simulink model "QAM16"  (R2024a)
settings: Solver=ode45  StartTime=0.0  StopTime=5000  RelTol=1e-3  EnableMultiTasking=on
PreLoadFcn:
  | QAM16_PreLoadFcn
values from neighbouring files (symbols this model uses):
  chan = [1+j*0.1 .2 j*0.2 0 0 0 0 0 0 0]    [QAM16_PreLoadFcn.m]
  hh = sinc(-3:.25:3)    [QAM16_PreLoadFcn.m]
  k = 9    [QAM16_PreLoadFcn.m]
  k_i0 = (4*theta_0*theta_0)/(1+2*eta*theta_0+theta_0*theta_0)    [QAM16_PreLoadFcn.m]
  k_p0 = (4*eta*theta_0)/(1+2*eta*theta_0+theta_0*theta_0)    [QAM16_PreLoadFcn.m]
  mu = 0.004    [QAM16_PreLoadFcn.m]
undefined symbols (not defined in the file or in its folder): j, QAM, S, vsva2197, xcvc1902, xlipgetpartsetting
libraries: hdlBasic x260, dspmlti4 x2, hdlUtilities x1, hdlDSPIP x1, simulink x1, vmcUtilities x1
(part 2 of 3)

== system QAM16/DUT/Carrier Recovery/DPLL Loop Filter ==
  phs_err : Inport
  KI : hdlBasic/Constant  Priority=5  const=k_i0  gui_display_data_type=Fixed-point  arith_type=Signed (2's comp)  n_bits=16  bin_pt=15  preci_type=Single  exp_width=8  frac_width=24  explicit_period=on  period=4  XmcBlockStatus=1  maskContainerNames=tabcontainer1  block_type=constant  block_config=sysgen:Constant_config
  KP : hdlBasic/Constant  Priority=5  const=k_p0  gui_display_data_type=Fixed-point  arith_type=Signed (2's comp)  n_bits=16  bin_pt=15  preci_type=Single  exp_width=8  frac_width=24  explicit_period=on  period=4  XmcBlockStatus=1  maskContainerNames=tabcontainer1  block_type=constant  block_config=sysgen:Constant_config
  MPY KI : hdlBasic/Mult  precision=User Defined  arith_type="Signed  (2's comp)"  n_bits=32  bin_pt=28  quantization=Truncate  overflow=Wrap  en=off  latency=0  opt_float=off  fp_mult_usage=No Usage  use_behavioral_HDL=off  opt=Speed  use_embedded=on  optimum_pipeline=off  pipeline=off  use_rpm=off  placement_style=Rectangular shape  XmcBlockStatus=1  maskContainerNames=group1  block_type=mult  block_config=sysgen:Mult_config  block_width=598  block_height=876
  MPY KP : hdlBasic/Mult  precision=User Defined  arith_type="Signed  (2's comp)"  n_bits=32  bin_pt=28  quantization=Truncate  overflow=Wrap  en=off  latency=0  opt_float=off  fp_mult_usage=No Usage  use_behavioral_HDL=off  opt=Speed  use_embedded=on  optimum_pipeline=off  pipeline=off  use_rpm=off  placement_style=Rectangular shape  XmcBlockStatus=1  maskContainerNames=group1  block_type=mult  block_config=sysgen:Mult_config  block_width=598  block_height=876
  addsub : hdlBasic/AddSub  mode=Addition  use_carryin=off  use_carryout=off  en=off  latency=0  precision=User Defined  arith_type=Unsigned  n_bits=10  bin_pt=10  quantization=Truncate  overflow=Wrap  use_behavioral_HDL=on  hw_selection=Fabric  pipelined=off  use_rpm=off  XmcBlockStatus=1  maskContainerNames=tabcontainer1  block_type=addsub  block_config=sysgen:Addsub_config
  addsub1 : hdlBasic/AddSub  mode=Addition  use_carryin=off  use_carryout=off  en=off  latency=0  precision=User Defined  arith_type="Signed  (2's comp)"  n_bits=32  bin_pt=28  quantization="Round  (unbiased: +/- Inf)"  overflow=Wrap  use_behavioral_HDL=on  hw_selection=Fabric  pipelined=off  use_rpm=off  XmcBlockStatus=1  maskContainerNames=tabcontainer1  block_type=addsub  block_config=sysgen:Addsub_config
  register : hdlBasic/Register  init=0  rst=off  en=off  XmcBlockStatus=1  maskContainerNames=tabcontainer1  block_type=register  block_config=sysgen:Register_config
  y : Outport  VectorParamsAs1DForOutWhenUnconnected=off
  wires:
  KI/1 -> MPY KI/2
  KP/1 -> MPY KP/2
  MPY KI/1 -> addsub1/1
  phs_err/1 -> MPY KI/1, MPY KP/1
  register/1 -> addsub1/2
  addsub1/1 -> addsub/2, register/1
  MPY KP/1 -> addsub/1
  addsub/1 -> y/1

== system QAM16/DUT/Carrier Recovery/Phase Detector ==
  note: The slicer circuit consistis primarily of several
      | comparators and a small look-up table.
  note: The arctangent operation is performed using
      | a custom CORDIC processor.
  I_in : Inport
  Q_in : Inport  Port=2
  Constant : hdlBasic/Constant  const=0  gui_display_data_type=Fixed-point  arith_type=Signed (2's comp)  n_bits=1  bin_pt=0  preci_type=Single  exp_width=8  frac_width=24  explicit_period=off  period=1  XmcBlockStatus=1  maskContainerNames=tabcontainer1  block_type=constant  block_config=sysgen:Constant_config
  Cordic : Subsystem
  NegB_Cmplx Mult : Subsystem
  Slicer : Subsystem
  Terminator : Terminator
  Terminator1 : Terminator
  det_I : Outport  VectorParamsAs1DForOutWhenUnconnected=off
  det_Q : Outport  Port=2  VectorParamsAs1DForOutWhenUnconnected=off
  phs_err : Outport  Port=3  VectorParamsAs1DForOutWhenUnconnected=off
  wires:
  NegB_Cmplx Mult/1(p_r) -> Cordic/1(x)
  Cordic/3(z_n) -> phs_err/1
  Constant/1 -> Cordic/3(z)
  Cordic/1(x_n) -> Terminator/1
  Cordic/2(y_n) -> Terminator1/1
  NegB_Cmplx Mult/2(p_i) -> Cordic/2(y)
  Slicer/2(det_Q) -> NegB_Cmplx Mult/2(a_i), det_Q/1
  Slicer/1(det_ I) -> NegB_Cmplx Mult/1(a_r), det_I/1
  Q_in/1 -> Slicer/2(Q_in), NegB_Cmplx Mult/4(b_i)
  I_in/1 -> Slicer/1(I_in), NegB_Cmplx Mult/3(b_r)

== system QAM16/16-QAM Data Shaping & Interpolation/QAM16 Source/QAM16 - I/Random Integer Generator ==
  Rounding Function : Rounding  Operator=round
  Uniform Random Number : UniformRandomNumber  Minimum=-0.49  Maximum=M-1 + 0.49  Seed=seed  SampleTime=Ts
  Out1 : Outport  VectorParamsAs1DForOutWhenUnconnected=off
  wires:
  Uniform Random Number/1 -> Rounding Function/1
  Rounding Function/1 -> Out1/1

== system QAM16/16-QAM Data Shaping & Interpolation/QAM16 Source/QAM16 -Q/Random Integer Generator ==
  Rounding Function : Rounding  Operator=round
  Uniform Random Number : UniformRandomNumber  Minimum=-0.49  Maximum=M-1 + 0.49  Seed=seed  SampleTime=Ts
  Out1 : Outport  VectorParamsAs1DForOutWhenUnconnected=off
  wires:
  Uniform Random Number/1 -> Rounding Function/1
  Rounding Function/1 -> Out1/1

== system QAM16/DUT/Adaptive Equalizer/ALU/PE0 ==
  note: The LMS error is used in conjunction with
      | delayed input data to update the filter
      | coefficient values.
  note: The LMS filter coefficients and current input
      | data samples are presented to the MAC FIR.
  note: Each LMS and FIR have their own local copy of the complex channel data. The reason is hardware
      | performance related, and in particular associated with the desire to pipeline the design to achieve
      | a suitable clock frequency. The memory systems in the FIR and LMS processors are skewed in
      | time with respect to each other. This effectively decouples the processes and permits the filter
      | and LMS engines to be heavily pipelined.
  x_r : Inport
  x_i : Inport  Port=2
  e_I : Inport  Port=3
  e_Q : Inport  Port=4
  Delay3 : hdlBasic/Delay  rst=off  en=off  latency=k  reg_retiming=off  XmcBlockStatus=1  maskContainerNames=group1  block_type=delay  block_config=sysgen:Delay_config
  Delay4 : hdlBasic/Delay  rst=off  en=off  latency=k  reg_retiming=off  XmcBlockStatus=1  maskContainerNames=group1  block_type=delay  block_config=sysgen:Delay_config
  Gateway Out : hdlBasic/Gateway Out  inherit_from_input=off  bool_to_boolean=off  hdl_port=off  rows=1  columns=1  UseAsDAC=off  DACChannel='1'  interface=None  automatic_assignment=on  address_offset=hex2dec('00')  intf_name=''  intf_description=''  timing_constraint=None  locs_specified=off  LOCs={}  io_standard={}  XmcBlockStatus=1  maskContainerNames=group4  block_type=gatewayout  block_config=sysgen:gateway_out_config  block_width_w=590  block_height_w=620  block_width=620  block_height=750
  Gateway Out1 : hdlBasic/Gateway Out  inherit_from_input=off  bool_to_boolean=off  hdl_port=off  rows=1  columns=1  UseAsDAC=off  DACChannel='1'  interface=None  automatic_assignment=on  address_offset=hex2dec('00')  intf_name=''  intf_description=''  timing_constraint=None  locs_specified=off  LOCs={}  io_standard={}  XmcBlockStatus=1  maskContainerNames=group4  block_type=gatewayout  block_config=sysgen:gateway_out_config  block_width_w=590  block_height_w=620  block_width=620  block_height=750
  LMS Update : Subsystem
  MAC FIR : Subsystem
  Real-Imag to Complex1 : RealImagToComplex
  d_r : Outport  VectorParamsAs1DForOutWhenUnconnected=off
  d_i : Outport  Port=2  VectorParamsAs1DForOutWhenUnconnected=off
  coef : Outport  Port=3  VectorParamsAs1DForOutWhenUnconnected=off
  wires:
  x_r/1 -> Delay3/1, MAC FIR/1(x_r)
  x_i/1 -> Delay4/1, MAC FIR/2(x_i)
  e_I/1 -> LMS Update/3(err_r)
  e_Q/1 -> LMS Update/4(err_i)
  Delay3/1 -> LMS Update/1(x_I)
  Delay4/1 -> LMS Update/2(x_Q)
  MAC FIR/1(y_r) -> d_r/1
  MAC FIR/2(y_i) -> d_i/1
  Gateway Out/1 -> Real-Imag to Complex1/1
  Gateway Out1/1 -> Real-Imag to Complex1/2
  Real-Imag to Complex1/1 -> coef/1
  LMS Update/2(coef_i) -> MAC FIR/4(coef_i), Gateway Out1/1
  LMS Update/1(coef_r) -> MAC FIR/3(coef_r), Gateway Out/1

== system QAM16/DUT/Adaptive Equalizer/ALU/PE1 ==
  x_r : Inport
  x_i : Inport  Port=2
  e_I : Inport  Port=3
  e_Q : Inport  Port=4
  Delay1 : hdlBasic/Delay  rst=off  en=off  latency=k  reg_retiming=off  XmcBlockStatus=1  maskContainerNames=group1  block_type=delay  block_config=sysgen:Delay_config
  Delay2 : hdlBasic/Delay  rst=off  en=off  latency=k  reg_retiming=off  XmcBlockStatus=1  maskContainerNames=group1  block_type=delay  block_config=sysgen:Delay_config
  Gateway Out2 : hdlBasic/Gateway Out  inherit_from_input=off  bool_to_boolean=off  hdl_port=off  rows=1  columns=1  UseAsDAC=off  DACChannel='1'  interface=None  automatic_assignment=on  address_offset=hex2dec('00')  intf_name=''  intf_description=''  timing_constraint=None  locs_specified=off  LOCs={}  io_standard={}  XmcBlockStatus=1  maskContainerNames=group4  block_type=gatewayout  block_config=sysgen:gateway_out_config  block_width_w=590  block_height_w=620  block_width=620  block_height=750
  Gateway Out3 : hdlBasic/Gateway Out  inherit_from_input=off  bool_to_boolean=off  hdl_port=off  rows=1  columns=1  UseAsDAC=off  DACChannel='1'  interface=None  automatic_assignment=on  address_offset=hex2dec('00')  intf_name=''  intf_description=''  timing_constraint=None  locs_specified=off  LOCs={}  io_standard={}  XmcBlockStatus=1  maskContainerNames=group4  block_type=gatewayout  block_config=sysgen:gateway_out_config  block_width_w=590  block_height_w=620  block_width=620  block_height=750
  LMS Update : Subsystem
  MAC FIR : Subsystem
  Real-Imag to Complex2 : RealImagToComplex
  d_r : Outport  VectorParamsAs1DForOutWhenUnconnected=off
  d_i : Outport  Port=2  VectorParamsAs1DForOutWhenUnconnected=off
  coef : Outport  Port=3  VectorParamsAs1DForOutWhenUnconnected=off
  wires:
  Gateway Out2/1 -> Real-Imag to Complex2/1
  Gateway Out3/1 -> Real-Imag to Complex2/2
  Real-Imag to Complex2/1 -> coef/1
  Delay2/1 -> LMS Update/2(x_Q)
  Delay1/1 -> LMS Update/1(x_I)
  LMS Update/1(coef_r) -> MAC FIR/3(coef_r), Gateway Out2/1
  LMS Update/2(coef_i) -> MAC FIR/4(coef_i), Gateway Out3/1
  MAC FIR/1(y_r) -> d_r/1
  MAC FIR/2(y_i) -> d_i/1
  e_Q/1 -> LMS Update/4(err_i)
  e_I/1 -> LMS Update/3(err_r)
  x_i/1 -> Delay2/1, MAC FIR/2(x_i)
  x_r/1 -> Delay1/1, MAC FIR/1(x_r)

== system QAM16/DUT/Carrier Recovery/Phase Detector/Cordic ==
  x : Inport
  y : Inport  Port=2
  z : Inport  Port=3
  Cordic Fine Angle PE : Subsystem
  Quadrant Correct : Subsystem
  Quadrant Map : Subsystem
  x_n : Outport  VectorParamsAs1DForOutWhenUnconnected=off
  y_n : Outport  Port=2  VectorParamsAs1DForOutWhenUnconnected=off
  z_n : Outport  Port=3  VectorParamsAs1DForOutWhenUnconnected=off
  wires:
  Cordic Fine Angle PE/1(x_n) -> x_n/1
  Cordic Fine Angle PE/2(y_n) -> y_n/1
  Cordic Fine Angle PE/3(z_n) -> Quadrant Correct/1(z_in)
  y/1 -> Quadrant Map/2(y)
  x/1 -> Quadrant Map/1(x)
  Quadrant Map/2(y_map) -> Cordic Fine Angle PE/2(y_0)
  Quadrant Map/1(x_map) -> Cordic Fine Angle PE/1(x_0)
  Quadrant Correct/1(z_out) -> z_n/1
  Quadrant Map/4(z_mux_sel) -> Quadrant Correct/3(z_mux_sel)
  Quadrant Map/3(" PI:2_add:sub") -> Quadrant Correct/2(pi:2_add:sub)
  z/1 -> Cordic Fine Angle PE/3(z_0)

== system QAM16/DUT/Carrier Recovery/Phase Detector/NegB_Cmplx Mult ==
  a_r : Inport
  a_i : Inport  Port=2
  b_r : Inport  Port=3
  b_i : Inport  Port=4
  AddSub : hdlBasic/AddSub  mode=Addition  use_carryin=off  use_carryout=off  en=off  latency=0  precision=User Defined  arith_type="Signed  (2's comp)"  n_bits=lms_mult_post_add_ni  bin_pt=lms_mult_post_add_nf  quantization=Truncate  overflow=Wrap  use_behavioral_HDL=on  hw_selection=Fabric  pipelined=off  use_rpm=on  XmcBlockStatus=1  maskContainerNames=tabcontainer1  block_type=addsub  block_config=sysgen:Addsub_config
  AddSub1 : hdlBasic/AddSub  mode=Subtraction  use_carryin=off  use_carryout=off  en=off  latency=0  precision=User Defined  arith_type="Signed  (2's comp)"  n_bits=lms_mult_post_add_ni  bin_pt=lms_mult_post_add_nf  quantization=Truncate  overflow=Wrap  use_behavioral_HDL=on  hw_selection=Fabric  pipelined=off  use_rpm=on  XmcBlockStatus=1  maskContainerNames=tabcontainer1  block_type=addsub  block_config=sysgen:Addsub_config
  Mult{1..4} (4 alike) : hdlBasic/Mult  precision=User Defined  arith_type="Signed  (2's comp)"  n_bits=lms_mult_ni  bin_pt=lms_mult_nf  quantization=Truncate  overflow=Wrap  en=off  latency=0  opt_float=off  fp_mult_usage=No Usage  use_behavioral_HDL=off  opt=Speed  use_embedded=on  optimum_pipeline=off  pipeline=off  use_rpm=on  placement_style=Rectangular shape  XmcBlockStatus=1  maskContainerNames=group1  block_type=mult  block_config=sysgen:Mult_config  block_width=598  block_height=876
  p_r : Outport  VectorParamsAs1DForOutWhenUnconnected=off
  p_i : Outport  Port=2  VectorParamsAs1DForOutWhenUnconnected=off
  wires:
  Mult4/1 -> AddSub/1
  a_i/1 -> Mult1/1, Mult3/2
  b_r/1 -> Mult4/2, Mult3/1
  b_i/1 -> Mult1/2, Mult2/2
  a_r/1 -> Mult4/1, Mult2/1
  Mult1/1 -> AddSub/2
  Mult2/1 -> AddSub1/1
  Mult3/1 -> AddSub1/2
  AddSub/1 -> p_r/1
  AddSub1/1 -> p_i/1

== system QAM16/DUT/Carrier Recovery/Phase Detector/Slicer ==
  I_in : Inport
  Q_in : Inport  Port=2
  I Map : Subsystem
  Q Map : Subsystem
  det_ I : Outport  VectorParamsAs1DForOutWhenUnconnected=off
  det_Q : Outport  Port=2  VectorParamsAs1DForOutWhenUnconnected=off
  wires:
  Q Map/1(det) -> det_Q/1
  I Map/1(det) -> det_ I/1
  I_in/1 -> I Map/1(x_n)
  Q_in/1 -> Q Map/1(x_n)

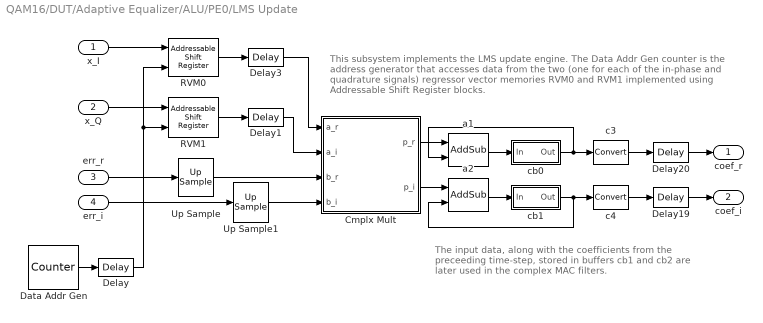
== system QAM16/DUT/Adaptive Equalizer/ALU/PE0/LMS Update ==
  note: This subsystem implements the LMS update engine. The Data Addr Gen
      | counter is the address generator that accesses data from the two (one for each of the
      | in-phase and quadrature signals) regressor vector memories RVM0 and RVM1
      | implemented using Addressable Shift Register blocks.
  note: The input data, along with the coefficients from the
      | preceeding time-step, stored in buffers cb1 and cb2
      | are later used in the complex MAC filters.
  x_I : Inport
  x_Q : Inport  Port=2
  err_r : Inport  Port=3
  err_i : Inport  Port=4
  Cmplx Mult : Subsystem
  Data Addr Gen : hdlBasic/Counter  cnt_type=Count limited  cnt_to=3  operation=Up  start_count=0  cnt_by_val=1  arith_type=Unsigned  n_bits=2  bin_pt=0  load_pin=off  rst=off  en=off  explicit_period=Explicit  period=T  use_behavioral_HDL=off  implementation=Fabric  use_rpm=off  XmcBlockStatus=1  maskContainerNames=group1  block_type=counter  block_config=sysgen:Counter_config  block_width=531  block_height=1023
  Delay : hdlBasic/Delay  rst=off  en=off  latency=1  reg_retiming=off  XmcBlockStatus=1  maskContainerNames=group1  block_type=delay  block_config=sysgen:Delay_config
  Delay1 : hdlBasic/Delay  rst=off  en=off  latency=3  reg_retiming=off  XmcBlockStatus=1  maskContainerNames=group1  block_type=delay  block_config=sysgen:Delay_config
  Delay19 : hdlBasic/Delay  rst=off  en=off  latency=6  reg_retiming=off  XmcBlockStatus=1  maskContainerNames=group1  block_type=delay  block_config=sysgen:Delay_config
  Delay20 : hdlBasic/Delay  rst=off  en=off  latency=6  reg_retiming=off  XmcBlockStatus=1  maskContainerNames=group1  block_type=delay  block_config=sysgen:Delay_config
  Delay3 : hdlBasic/Delay  rst=off  en=off  latency=3  reg_retiming=off  XmcBlockStatus=1  maskContainerNames=group1  block_type=delay  block_config=sysgen:Delay_config
  RVM0 : hdlBasic/Addressable Shift Register  infer_latency=off  depth=4  initVector=[0]  en=off  use_behavioral_HDL=off  Optimization=Resource  use_rpm=off  XmcBlockStatus=1  maskContainerNames=group1  block_type=addrsr  block_config=sysgen:Addrsr_config
  RVM1 : hdlBasic/Addressable Shift Register  infer_latency=off  depth=4  initVector=[0]  en=off  use_behavioral_HDL=off  Optimization=Resource  use_rpm=off  XmcBlockStatus=1  maskContainerNames=group1  block_type=addrsr  block_config=sysgen:Addrsr_config
  Up Sample : hdlBasic/Up Sample  sample_ratio=4  copy_samples=on  en=off  latency=0  XmcBlockStatus=1  maskContainerNames=group1  block_type=usamp  block_config=sysgen:Upsample_config
  Up Sample1 : hdlBasic/Up Sample  sample_ratio=4  copy_samples=on  en=off  latency=0  XmcBlockStatus=1  maskContainerNames=group1  block_type=usamp  block_config=sysgen:Upsample_config
  a1 : hdlBasic/AddSub  mode=Addition  use_carryin=off  use_carryout=off  en=off  latency=0  precision=User Defined  arith_type="Signed  (2's comp)"  n_bits=lms_acc_ni  bin_pt=lms_acc_nf  quantization="Round  (unbiased: +/- Inf)"  overflow=Wrap  use_behavioral_HDL=on  hw_selection=Fabric  pipelined=off  use_rpm=on  XmcBlockStatus=1  maskContainerNames=tabcontainer1  block_type=addsub  block_config=sysgen:Addsub_config
  a2 : hdlBasic/AddSub  mode=Addition  use_carryin=off  use_carryout=off  en=off  latency=0  precision=User Defined  arith_type="Signed  (2's comp)"  n_bits=lms_acc_ni  bin_pt=lms_acc_nf  quantization="Round  (unbiased: +/- Inf)"  overflow=Wrap  use_behavioral_HDL=on  hw_selection=Fabric  pipelined=off  use_rpm=on  XmcBlockStatus=1  maskContainerNames=tabcontainer1  block_type=addsub  block_config=sysgen:Addsub_config
  c3 : hdlBasic/Convert  gui_display_data_type=Fixed-point  arith_type=Signed (2's comp)  n_bits=coeff_ni  bin_pt=coeff_nf  float_type=Single  exp_bits=8  fraction_bits=24  quantization="Round  (unbiased: +/- Inf)"  overflow=Wrap  en=off  latency=0  pipeline=off  XmcBlockStatus=1  maskContainerNames=group2  block_type=convert  block_config=sysgen:Convert_config  block_width=595  block_height=885
  c4 : hdlBasic/Convert  gui_display_data_type=Fixed-point  arith_type=Signed (2's comp)  n_bits=coeff_ni  bin_pt=coeff_nf  float_type=Single  exp_bits=8  fraction_bits=24  quantization="Round  (unbiased: +/- Inf)"  overflow=Wrap  en=off  latency=0  pipeline=off  XmcBlockStatus=1  maskContainerNames=group2  block_type=convert  block_config=sysgen:Convert_config  block_width=595  block_height=885
  cb0 : Subsystem
  cb1 : Subsystem
  coef_r : Outport  VectorParamsAs1DForOutWhenUnconnected=off
  coef_i : Outport  Port=2  VectorParamsAs1DForOutWhenUnconnected=off
  wires:
  x_I/1 -> RVM0/1
  RVM0/1 -> Delay3/1
  x_Q/1 -> RVM1/1
  RVM1/1 -> Delay1/1
  Delay3/1 -> Cmplx Mult/1(a_r)
  Delay1/1 -> Cmplx Mult/2(a_i)
  a1/1 -> cb0/1(In)
  a2/1 -> cb1/1(In)
  cb0/1(Out) -> c3/1, a1/2
  cb1/1(Out) -> c4/1, a2/2
  err_r/1 -> Up Sample/1
  err_i/1 -> Up Sample1/1
  Up Sample/1 -> Cmplx Mult/3(b_r)
  Up Sample1/1 -> Cmplx Mult/4(b_i)
  Data Addr Gen/1 -> Delay/1
  Delay/1 -> RVM1/2, RVM0/2
  c3/1 -> Delay20/1
  c4/1 -> Delay19/1
  Delay19/1 -> coef_i/1
  Delay20/1 -> coef_r/1
  Cmplx Mult/1(p_r) -> a1/1
  Cmplx Mult/2(p_i) -> a2/1

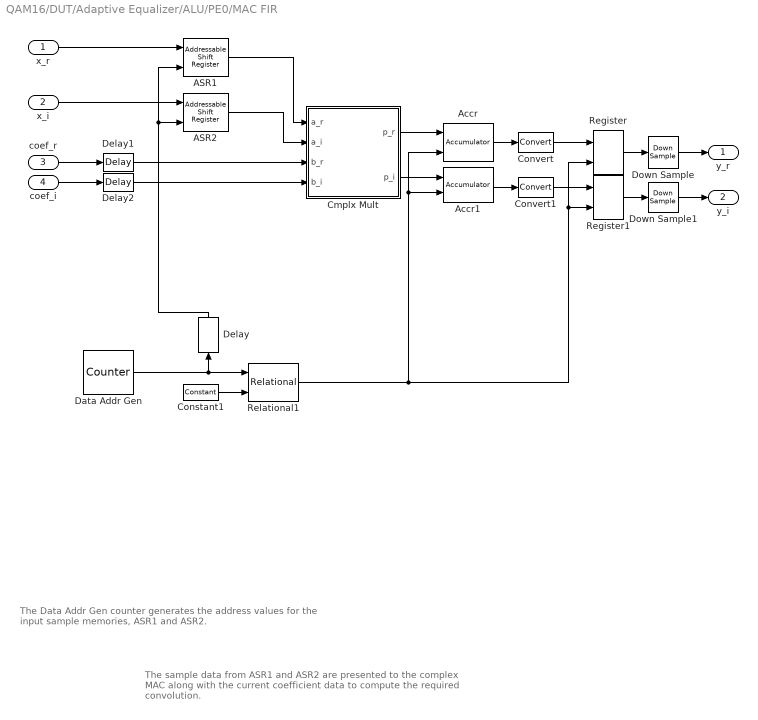
== system QAM16/DUT/Adaptive Equalizer/ALU/PE0/MAC FIR ==
  note: The sample data from ASR1 and ASR2 are presented to the
      | complex MAC along with the current coefficient  data to compute
      | the required convolution.
  note: The Data Addr Gen counter generates the address values for
      | the input sample memories, ASR1 and ASR2.
  x_r : Inport
  x_i : Inport  Port=2
  coef_r : Inport  Port=3
  coef_i : Inport  Port=4
  ASR1 : hdlBasic/Addressable Shift Register  infer_latency=off  depth=4  initVector=[0]  en=off  use_behavioral_HDL=off  Optimization=Resource  use_rpm=off  XmcBlockStatus=1  maskContainerNames=group1  block_type=addrsr  block_config=sysgen:Addrsr_config
  ASR2 : hdlBasic/Addressable Shift Register  infer_latency=off  depth=4  initVector=[0]  en=off  use_behavioral_HDL=off  Optimization=Resource  use_rpm=off  XmcBlockStatus=1  maskContainerNames=group1  block_type=addrsr  block_config=sysgen:Addrsr_config
  Accr : hdlBasic/Accumulator  operation=Add  n_bits=46  overflow=Wrap  scale=1  rst=on  hasbypass=on  en=off  latency=1  msb_inp=100  msb=100  lsb=-100  use_behavioral_HDL=on  implementation=Fabric  XmcBlockStatus=1  maskContainerNames=group3  block_type=accum  block_config=sysgen:Accum_config  block_width=566  block_height=845
  Accr1 : hdlBasic/Accumulator  operation=Add  n_bits=46  overflow=Wrap  scale=1  rst=on  hasbypass=on  en=off  latency=1  msb_inp=100  msb=100  lsb=-100  use_behavioral_HDL=on  implementation=Fabric  XmcBlockStatus=1  maskContainerNames=group3  block_type=accum  block_config=sysgen:Accum_config  block_width=566  block_height=845
  Cmplx Mult : Subsystem
  Constant1 : hdlBasic/Constant  const=0  gui_display_data_type=Fixed-point  arith_type=Unsigned  n_bits=1  bin_pt=0  preci_type=Single  exp_width=8  frac_width=24  explicit_period=on  period=T  XmcBlockStatus=1  maskContainerNames=tabcontainer1  block_type=constant  block_config=sysgen:Constant_config
  Convert : hdlBasic/Convert  gui_display_data_type=Fixed-point  arith_type=Signed (2's comp)  n_bits=24  bin_pt=20  float_type=Single  exp_bits=8  fraction_bits=24  quantization="Round  (unbiased: +/- Inf)"  overflow=Wrap  en=off  latency=0  pipeline=off  XmcBlockStatus=1  maskContainerNames=group2  block_type=convert  block_config=sysgen:Convert_config  block_width=595  block_height=885
  Convert1 : hdlBasic/Convert  gui_display_data_type=Fixed-point  arith_type=Signed (2's comp)  n_bits=24  bin_pt=20  float_type=Single  exp_bits=8  fraction_bits=24  quantization="Round  (unbiased: +/- Inf)"  overflow=Wrap  en=off  latency=0  pipeline=off  XmcBlockStatus=1  maskContainerNames=group2  block_type=convert  block_config=sysgen:Convert_config  block_width=595  block_height=885
  Data Addr Gen : hdlBasic/Counter  cnt_type=Count limited  cnt_to=3  operation=Up  start_count=0  cnt_by_val=1  arith_type=Unsigned  n_bits=2  bin_pt=0  load_pin=off  rst=off  en=off  explicit_period=Explicit  period=T  use_behavioral_HDL=off  implementation=Fabric  use_rpm=off  XmcBlockStatus=1  maskContainerNames=group1  block_type=counter  block_config=sysgen:Counter_config  block_width=531  block_height=1023
  Delay : hdlBasic/Delay  rst=off  en=off  latency=1  reg_retiming=off  XmcBlockStatus=1  maskContainerNames=group1  block_type=delay  block_config=sysgen:Delay_config
  Delay1 : hdlBasic/Delay  rst=off  en=off  latency=1  reg_retiming=off  XmcBlockStatus=1  maskContainerNames=group1  block_type=delay  block_config=sysgen:Delay_config
  Delay2 : hdlBasic/Delay  rst=off  en=off  latency=1  reg_retiming=off  XmcBlockStatus=1  maskContainerNames=group1  block_type=delay  block_config=sysgen:Delay_config
  Down Sample : hdlBasic/Down Sample  sample_ratio=4  sample_phase="Last Value of Frame  (most efficient)"  en=off  rst=off  latency=1  XmcBlockStatus=1  maskContainerNames=group1  block_type=dsamp  block_config=sysgen:Downsample_config
  Down Sample1 : hdlBasic/Down Sample  sample_ratio=4  sample_phase="Last Value of Frame  (most efficient)"  en=off  rst=off  latency=1  XmcBlockStatus=1  maskContainerNames=group1  block_type=dsamp  block_config=sysgen:Downsample_config
  Register : hdlBasic/Register  init=0  rst=off  en=on  XmcBlockStatus=1  maskContainerNames=tabcontainer1  block_type=register  block_config=sysgen:Register_config
  Register1 : hdlBasic/Register  init=0  rst=off  en=on  XmcBlockStatus=1  maskContainerNames=tabcontainer1  block_type=register  block_config=sysgen:Register_config
  Relational1 : hdlBasic/Relational  mode=a=b  op_type=Bool  en=off  latency=7  XmcBlockStatus=1  maskContainerNames=tabcontainer1  block_type=relational  block_config=sysgen:Relational_config
  y_r : Outport  VectorParamsAs1DForOutWhenUnconnected=off
  y_i : Outport  Port=2  VectorParamsAs1DForOutWhenUnconnected=off
  wires:
  Delay/1 -> ASR1/2, ASR2/2
  x_r/1 -> ASR1/1
  ASR1/1 -> Cmplx Mult/1(a_r)
  x_i/1 -> ASR2/1
  ASR2/1 -> Cmplx Mult/2(a_i)
  coef_r/1 -> Delay1/1
  coef_i/1 -> Delay2/1
  Delay2/1 -> Cmplx Mult/4(b_i)
  Delay1/1 -> Cmplx Mult/3(b_r)
  Accr/1 -> Convert/1
  Cmplx Mult/1(p_r) -> Accr/1
  Cmplx Mult/2(p_i) -> Accr1/1
  Accr1/1 -> Convert1/1
  Relational1/1 -> Register/2, Register1/2, Accr/2, Accr1/2
  Register/1 -> Down Sample/1
  Register1/1 -> Down Sample1/1
  Convert/1 -> Register/1
  Convert1/1 -> Register1/1
  Down Sample/1 -> y_r/1
  Down Sample1/1 -> y_i/1
  Data Addr Gen/1 -> Relational1/1, Delay/1
  Constant1/1 -> Relational1/2

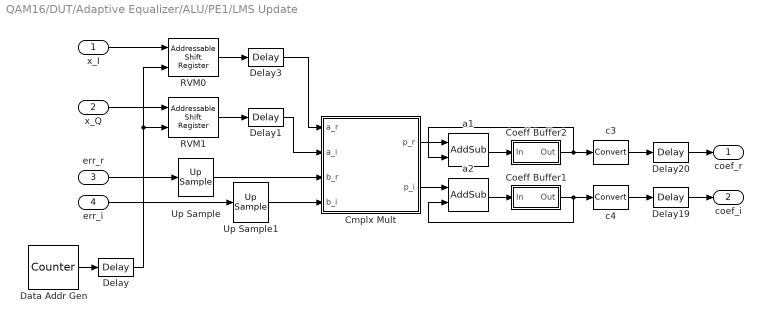
== system QAM16/DUT/Adaptive Equalizer/ALU/PE1/LMS Update ==
  x_I : Inport
  x_Q : Inport  Port=2
  err_r : Inport  Port=3
  err_i : Inport  Port=4
  Cmplx Mult : Subsystem
  Coeff Buffer1 : Subsystem
  Coeff Buffer2 : Subsystem
  Data Addr Gen : hdlBasic/Counter  cnt_type=Count limited  cnt_to=3  operation=Up  start_count=0  cnt_by_val=1  arith_type=Unsigned  n_bits=2  bin_pt=0  load_pin=off  rst=off  en=off  explicit_period=Explicit  period=T  use_behavioral_HDL=off  implementation=Fabric  use_rpm=off  XmcBlockStatus=1  maskContainerNames=group1  block_type=counter  block_config=sysgen:Counter_config  block_width=531  block_height=1023
  Delay : hdlBasic/Delay  rst=off  en=off  latency=1  reg_retiming=off  XmcBlockStatus=1  maskContainerNames=group1  block_type=delay  block_config=sysgen:Delay_config
  Delay1 : hdlBasic/Delay  rst=off  en=off  latency=3  reg_retiming=off  XmcBlockStatus=1  maskContainerNames=group1  block_type=delay  block_config=sysgen:Delay_config
  Delay19 : hdlBasic/Delay  rst=off  en=off  latency=6  reg_retiming=off  XmcBlockStatus=1  maskContainerNames=group1  block_type=delay  block_config=sysgen:Delay_config
  Delay20 : hdlBasic/Delay  rst=off  en=off  latency=6  reg_retiming=off  XmcBlockStatus=1  maskContainerNames=group1  block_type=delay  block_config=sysgen:Delay_config
  Delay3 : hdlBasic/Delay  rst=off  en=off  latency=3  reg_retiming=off  XmcBlockStatus=1  maskContainerNames=group1  block_type=delay  block_config=sysgen:Delay_config
  RVM0 : hdlBasic/Addressable Shift Register  infer_latency=off  depth=4  initVector=[0]  en=off  use_behavioral_HDL=off  Optimization=Resource  use_rpm=off  XmcBlockStatus=1  maskContainerNames=group1  block_type=addrsr  block_config=sysgen:Addrsr_config
  RVM1 : hdlBasic/Addressable Shift Register  infer_latency=off  depth=4  initVector=[0]  en=off  use_behavioral_HDL=off  Optimization=Resource  use_rpm=off  XmcBlockStatus=1  maskContainerNames=group1  block_type=addrsr  block_config=sysgen:Addrsr_config
  Up Sample : hdlBasic/Up Sample  sample_ratio=4  copy_samples=on  en=off  latency=0  XmcBlockStatus=1  maskContainerNames=group1  block_type=usamp  block_config=sysgen:Upsample_config
  Up Sample1 : hdlBasic/Up Sample  sample_ratio=4  copy_samples=on  en=off  latency=0  XmcBlockStatus=1  maskContainerNames=group1  block_type=usamp  block_config=sysgen:Upsample_config
  a1 : hdlBasic/AddSub  mode=Addition  use_carryin=off  use_carryout=off  en=off  latency=0  precision=User Defined  arith_type="Signed  (2's comp)"  n_bits=lms_acc_ni  bin_pt=lms_acc_nf  quantization="Round  (unbiased: +/- Inf)"  overflow=Wrap  use_behavioral_HDL=on  hw_selection=Fabric  pipelined=off  use_rpm=on  XmcBlockStatus=1  maskContainerNames=tabcontainer1  block_type=addsub  block_config=sysgen:Addsub_config
  a2 : hdlBasic/AddSub  mode=Addition  use_carryin=off  use_carryout=off  en=off  latency=0  precision=User Defined  arith_type="Signed  (2's comp)"  n_bits=lms_acc_ni  bin_pt=lms_acc_nf  quantization="Round  (unbiased: +/- Inf)"  overflow=Wrap  use_behavioral_HDL=on  hw_selection=Fabric  pipelined=off  use_rpm=on  XmcBlockStatus=1  maskContainerNames=tabcontainer1  block_type=addsub  block_config=sysgen:Addsub_config
  c3 : hdlBasic/Convert  gui_display_data_type=Fixed-point  arith_type=Signed (2's comp)  n_bits=coeff_ni  bin_pt=coeff_nf  float_type=Single  exp_bits=8  fraction_bits=24  quantization="Round  (unbiased: +/- Inf)"  overflow=Wrap  en=off  latency=0  pipeline=off  XmcBlockStatus=1  maskContainerNames=group2  block_type=convert  block_config=sysgen:Convert_config  block_width=595  block_height=885
  c4 : hdlBasic/Convert  gui_display_data_type=Fixed-point  arith_type=Signed (2's comp)  n_bits=coeff_ni  bin_pt=coeff_nf  float_type=Single  exp_bits=8  fraction_bits=24  quantization="Round  (unbiased: +/- Inf)"  overflow=Wrap  en=off  latency=0  pipeline=off  XmcBlockStatus=1  maskContainerNames=group2  block_type=convert  block_config=sysgen:Convert_config  block_width=595  block_height=885
  coef_r : Outport  VectorParamsAs1DForOutWhenUnconnected=off
  coef_i : Outport  Port=2  VectorParamsAs1DForOutWhenUnconnected=off
  wires:
  x_I/1 -> RVM0/1
  RVM0/1 -> Delay3/1
  x_Q/1 -> RVM1/1
  RVM1/1 -> Delay1/1
  Delay3/1 -> Cmplx Mult/1(a_r)
  Delay1/1 -> Cmplx Mult/2(a_i)
  a1/1 -> Coeff Buffer2/1(In)
  a2/1 -> Coeff Buffer1/1(In)
  Coeff Buffer2/1(Out) -> c3/1, a1/2
  Coeff Buffer1/1(Out) -> c4/1, a2/2
  err_r/1 -> Up Sample/1
  err_i/1 -> Up Sample1/1
  Up Sample/1 -> Cmplx Mult/3(b_r)
  Up Sample1/1 -> Cmplx Mult/4(b_i)
  Data Addr Gen/1 -> Delay/1
  Delay/1 -> RVM1/2, RVM0/2
  c3/1 -> Delay20/1
  c4/1 -> Delay19/1
  Delay19/1 -> coef_i/1
  Delay20/1 -> coef_r/1
  Cmplx Mult/1(p_r) -> a1/1
  Cmplx Mult/2(p_i) -> a2/1

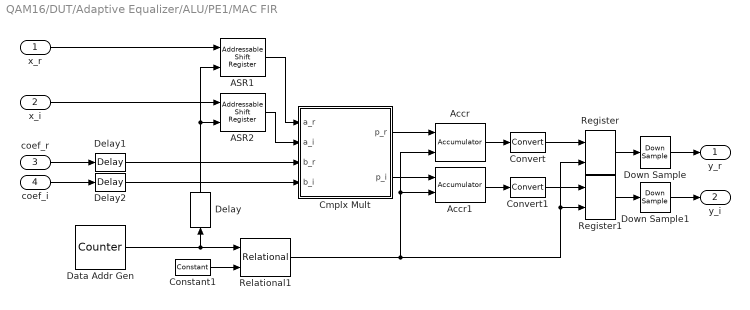
== system QAM16/DUT/Adaptive Equalizer/ALU/PE1/MAC FIR ==
  x_r : Inport
  x_i : Inport  Port=2
  coef_r : Inport  Port=3
  coef_i : Inport  Port=4
  ASR1 : hdlBasic/Addressable Shift Register  infer_latency=off  depth=4  initVector=[0]  en=off  use_behavioral_HDL=off  Optimization=Resource  use_rpm=off  XmcBlockStatus=1  maskContainerNames=group1  block_type=addrsr  block_config=sysgen:Addrsr_config
  ASR2 : hdlBasic/Addressable Shift Register  infer_latency=off  depth=4  initVector=[0]  en=off  use_behavioral_HDL=off  Optimization=Resource  use_rpm=off  XmcBlockStatus=1  maskContainerNames=group1  block_type=addrsr  block_config=sysgen:Addrsr_config
  Accr : hdlBasic/Accumulator  operation=Add  n_bits=46  overflow=Wrap  scale=1  rst=on  hasbypass=on  en=off  latency=1  msb_inp=100  msb=100  lsb=-100  use_behavioral_HDL=on  implementation=Fabric  XmcBlockStatus=1  maskContainerNames=group3  block_type=accum  block_config=sysgen:Accum_config  block_width=566  block_height=845
  Accr1 : hdlBasic/Accumulator  operation=Add  n_bits=46  overflow=Wrap  scale=1  rst=on  hasbypass=on  en=off  latency=1  msb_inp=100  msb=100  lsb=-100  use_behavioral_HDL=on  implementation=Fabric  XmcBlockStatus=1  maskContainerNames=group3  block_type=accum  block_config=sysgen:Accum_config  block_width=566  block_height=845
  Cmplx Mult : Subsystem
  Constant1 : hdlBasic/Constant  const=0  gui_display_data_type=Fixed-point  arith_type=Unsigned  n_bits=1  bin_pt=0  preci_type=Single  exp_width=8  frac_width=24  explicit_period=on  period=T  XmcBlockStatus=1  maskContainerNames=tabcontainer1  block_type=constant  block_config=sysgen:Constant_config
  Convert : hdlBasic/Convert  gui_display_data_type=Fixed-point  arith_type=Signed (2's comp)  n_bits=24  bin_pt=20  float_type=Single  exp_bits=8  fraction_bits=24  quantization="Round  (unbiased: +/- Inf)"  overflow=Wrap  en=off  latency=0  pipeline=off  XmcBlockStatus=1  maskContainerNames=group2  block_type=convert  block_config=sysgen:Convert_config  block_width=595  block_height=885
  Convert1 : hdlBasic/Convert  gui_display_data_type=Fixed-point  arith_type=Signed (2's comp)  n_bits=24  bin_pt=20  float_type=Single  exp_bits=8  fraction_bits=24  quantization="Round  (unbiased: +/- Inf)"  overflow=Wrap  en=off  latency=0  pipeline=off  XmcBlockStatus=1  maskContainerNames=group2  block_type=convert  block_config=sysgen:Convert_config  block_width=595  block_height=885
  Data Addr Gen : hdlBasic/Counter  cnt_type=Count limited  cnt_to=3  operation=Up  start_count=0  cnt_by_val=1  arith_type=Unsigned  n_bits=2  bin_pt=0  load_pin=off  rst=off  en=off  explicit_period=Explicit  period=T  use_behavioral_HDL=off  implementation=Fabric  use_rpm=off  XmcBlockStatus=1  maskContainerNames=group1  block_type=counter  block_config=sysgen:Counter_config  block_width=531  block_height=1023
  Delay : hdlBasic/Delay  rst=off  en=off  latency=1  reg_retiming=off  XmcBlockStatus=1  maskContainerNames=group1  block_type=delay  block_config=sysgen:Delay_config
  Delay1 : hdlBasic/Delay  rst=off  en=off  latency=1  reg_retiming=off  XmcBlockStatus=1  maskContainerNames=group1  block_type=delay  block_config=sysgen:Delay_config
  Delay2 : hdlBasic/Delay  rst=off  en=off  latency=1  reg_retiming=off  XmcBlockStatus=1  maskContainerNames=group1  block_type=delay  block_config=sysgen:Delay_config
  Down Sample : hdlBasic/Down Sample  sample_ratio=4  sample_phase="Last Value of Frame  (most efficient)"  en=off  rst=off  latency=1  XmcBlockStatus=1  maskContainerNames=group1  block_type=dsamp  block_config=sysgen:Downsample_config
  Down Sample1 : hdlBasic/Down Sample  sample_ratio=4  sample_phase="Last Value of Frame  (most efficient)"  en=off  rst=off  latency=1  XmcBlockStatus=1  maskContainerNames=group1  block_type=dsamp  block_config=sysgen:Downsample_config
  Register : hdlBasic/Register  init=0  rst=off  en=on  XmcBlockStatus=1  maskContainerNames=tabcontainer1  block_type=register  block_config=sysgen:Register_config
  Register1 : hdlBasic/Register  init=0  rst=off  en=on  XmcBlockStatus=1  maskContainerNames=tabcontainer1  block_type=register  block_config=sysgen:Register_config
  Relational1 : hdlBasic/Relational  mode=a=b  op_type=Bool  en=off  latency=7  XmcBlockStatus=1  maskContainerNames=tabcontainer1  block_type=relational  block_config=sysgen:Relational_config
  y_r : Outport  VectorParamsAs1DForOutWhenUnconnected=off
  y_i : Outport  Port=2  VectorParamsAs1DForOutWhenUnconnected=off
  wires:
  Delay/1 -> ASR1/2, ASR2/2
  x_r/1 -> ASR1/1
  ASR1/1 -> Cmplx Mult/1(a_r)
  x_i/1 -> ASR2/1
  ASR2/1 -> Cmplx Mult/2(a_i)
  coef_r/1 -> Delay1/1
  coef_i/1 -> Delay2/1
  Delay2/1 -> Cmplx Mult/4(b_i)
  Delay1/1 -> Cmplx Mult/3(b_r)
  Accr/1 -> Convert/1
  Cmplx Mult/1(p_r) -> Accr/1
  Cmplx Mult/2(p_i) -> Accr1/1
  Accr1/1 -> Convert1/1
  Relational1/1 -> Accr/2, Accr1/2, Register/2, Register1/2
  Register/1 -> Down Sample/1
  Register1/1 -> Down Sample1/1
  Convert/1 -> Register/1
  Convert1/1 -> Register1/1
  Down Sample/1 -> y_r/1
  Down Sample1/1 -> y_i/1
  Data Addr Gen/1 -> Relational1/1, Delay/1
  Constant1/1 -> Relational1/2

== system QAM16/DUT/Carrier Recovery/Phase Detector/Cordic/Cordic Fine Angle PE ==
  note: The CORDIC processor uses a fully unfolded architecture, using 5 iterations
      | and 11-bit precision input samples.  Bit-growth to the final output precision of
      | 16-bits is permitted.
  x_0 : Inport
  y_0 : Inport  Port=2
  z_0 : Inport  Port=3
  Cordic PE0 : Subsystem
  Cordic PE1 : Subsystem
  Cordic PE2 : Subsystem
  Cordic PE3 : Subsystem
  Cordic PE4 : Subsystem
  x_n : Outport  VectorParamsAs1DForOutWhenUnconnected=off
  y_n : Outport  Port=2  VectorParamsAs1DForOutWhenUnconnected=off
  z_n : Outport  Port=3  VectorParamsAs1DForOutWhenUnconnected=off
  wires:
  Cordic PE4/3(z) -> z_n/1
  Cordic PE4/2(y) -> y_n/1
  Cordic PE4/1(x) -> x_n/1
  Cordic PE2/3(z) -> Cordic PE3/3(z_n-1)
  Cordic PE2/2(y) -> Cordic PE3/2(y_n-1)
  Cordic PE2/1(x) -> Cordic PE3/1(x_n-1)
  Cordic PE1/3(z) -> Cordic PE2/3(z_n-1)
  Cordic PE1/2(y) -> Cordic PE2/2(y_n-1)
  Cordic PE1/1(x) -> Cordic PE2/1(x_n-1)
  Cordic PE0/3(z) -> Cordic PE1/3(z_n-1)
  Cordic PE0/2(y) -> Cordic PE1/2(y_n-1)
  Cordic PE0/1(x) -> Cordic PE1/1(x_n-1)
  z_0/1 -> Cordic PE0/3(z_n-1)
  y_0/1 -> Cordic PE0/2(y_n-1)
  x_0/1 -> Cordic PE0/1(x_n-1)
  Cordic PE3/1(x) -> Cordic PE4/1(x_n-1)
  Cordic PE3/2(y) -> Cordic PE4/2(y_n-1)
  Cordic PE3/3(z) -> Cordic PE4/3(z_n-1)

== system QAM16/DUT/Carrier Recovery/Phase Detector/Cordic/Quadrant Correct ==
  z_in : Inport
  pi:2_add:sub : Inport  Port=2
  z_mux_sel : Inport  Port=3
  AddSub1 : hdlBasic/AddSub  mode=Addition or Subtraction  use_carryin=off  use_carryout=off  en=off  latency=0  precision=User Defined  arith_type="Signed  (2's comp)"  n_bits=atan_nbits  bin_pt=atan_nbits_frac  quantization=Truncate  overflow=Wrap  use_behavioral_HDL=on  hw_selection=Fabric  pipelined=off  use_rpm=off  XmcBlockStatus=1  maskContainerNames=tabcontainer1  block_type=addsub  block_config=sysgen:Addsub_config
  Mux : hdlBasic/Mux  inputs=2  en=off  latency=0  precision=Full  arith_type="Signed  (2's comp)"  n_bits=8  bin_pt=2  quantization=Truncate  overflow=Wrap  XmcBlockStatus=1  maskContainerNames=tabcontainer1  block_type=mux  block_config=sysgen:Mux_config
  PI:2 : hdlBasic/Constant  const=pi/2  gui_display_data_type=Fixed-point  arith_type=Signed (2's comp)  n_bits=atan_nbits  bin_pt=atan_nbits_frac  preci_type=Single  exp_width=8  frac_width=24  explicit_period=off  period=1  XmcBlockStatus=1  maskContainerNames=tabcontainer1  block_type=constant  block_config=sysgen:Constant_config
  z_out : Outport  VectorParamsAs1DForOutWhenUnconnected=off
  wires:
  z_mux_sel/1 -> Mux/1
  AddSub1/1 -> Mux/3
  PI:2/1 -> AddSub1/2
  pi:2_add:sub/1 -> AddSub1/3
  Mux/1 -> z_out/1
  z_in/1 -> AddSub1/1, Mux/2

== system QAM16/DUT/Carrier Recovery/Phase Detector/Cordic/Quadrant Map ==
  x : Inport
  y : Inport  Port=2
  Concat : hdlBasic/Concat  num_inputs=2  XmcBlockStatus=1  maskContainerNames=group1  block_type=concat  block_config=sysgen:Concat_config
  Mux : hdlBasic/Mux  inputs=3  en=off  latency=0  precision=User Defined  arith_type="Signed  (2's comp)"  n_bits=cordic_pe_nbits_total  bin_pt=cordic_pe_nbits_frac  quantization=Truncate  overflow=Wrap  XmcBlockStatus=1  maskContainerNames=tabcontainer1  block_type=mux  block_config=sysgen:Mux_config
  Mux1 : hdlBasic/Mux  inputs=3  en=off  latency=0  precision=User Defined  arith_type="Signed  (2's comp)"  n_bits=cordic_pe_nbits_total  bin_pt=cordic_pe_nbits_frac  quantization=Truncate  overflow=Wrap  XmcBlockStatus=1  maskContainerNames=tabcontainer1  block_type=mux  block_config=sysgen:Mux_config
  Negate : hdlBasic/Negate  precision=User Defined  arith_type=Unsigned  n_bits=cordic_pe_nbits_total  bin_pt=cordic_pe_nbits_frac  quantization=Truncate  overflow=Wrap  en=off  latency=0  XmcBlockStatus=1  maskContainerNames=tabcontainer1  block_type=negate  block_config=sysgen:Negate_config
  Negate1 : hdlBasic/Negate  precision=User Defined  arith_type=Unsigned  n_bits=cordic_pe_nbits_total  bin_pt=cordic_pe_nbits_frac  quantization=Truncate  overflow=Wrap  en=off  latency=0  XmcBlockStatus=1  maskContainerNames=tabcontainer1  block_type=negate  block_config=sysgen:Negate_config
  ROM : hdlBasic/ROM  depth=4  initVector=[0 1 0 2]  distributed_mem=Distributed memory  rst=off  init_reg=0  en=off  latency=0  gui_display_data_type=Fixed-point  arith_type=Unsigned  n_bits=2  bin_pt=0  preci_type=Single  exp_width=8  frac_width=24  optimize=Area  use_rpm=off  simulation_type=fast_sim  XmcBlockStatus=1  maskContainerNames=tabcontainer1  block_type=sprom  block_config=sysgen:SPROM_config
  sgn(x) : hdlBasic/Slice  nbits=1  boolean_output=on  mode=Upper Bit Location + Width  bit1=0  base1=MSB of Input  bit0=0  base0=LSB of Input  XmcBlockStatus=1  maskContainerNames=group1  block_type=slice  block_config=sysgen:Slice_config
  sgn(y) : hdlBasic/Slice  nbits=1  boolean_output=on  mode=Upper Bit Location + Width  bit1=0  base1=MSB of Input  bit0=0  base0=LSB of Input  XmcBlockStatus=1  maskContainerNames=group1  block_type=slice  block_config=sysgen:Slice_config
  x_map : Outport  VectorParamsAs1DForOutWhenUnconnected=off
  y_map : Outport  Port=2  VectorParamsAs1DForOutWhenUnconnected=off
  " PI:2_add:sub" : Outport  Port=3  VectorParamsAs1DForOutWhenUnconnected=off
  z_mux_sel : Outport  Port=4  VectorParamsAs1DForOutWhenUnconnected=off
  wires:
  ROM/1 -> Mux1/1, Mux/1
  Concat/1 -> ROM/1
  sgn(x)/1 -> z_mux_sel/1, Concat/2
  sgn(y)/1 -> " PI:2_add:sub"/1, Concat/1
  Negate1/1 -> Mux/4
  Negate/1 -> Mux1/3
  Mux1/1 -> y_map/1
  Mux/1 -> x_map/1
  y/1 -> Negate1/1, Mux/3, Mux1/2, sgn(y)/1
  x/1 -> Negate/1, Mux1/4, sgn(x)/1, Mux/2

== system QAM16/DUT/Carrier Recovery/Phase Detector/Slicer/I Map ==
  x_n : Inport
  Concat : hdlBasic/Concat  num_inputs=2  XmcBlockStatus=1  maskContainerNames=group1  block_type=concat  block_config=sysgen:Concat_config
  Mux : hdlBasic/Mux  inputs=2  en=off  latency=0  precision=Full  arith_type="Signed  (2's comp)"  n_bits=8  bin_pt=2  quantization=Truncate  overflow=Wrap  XmcBlockStatus=1  maskContainerNames=tabcontainer1  block_type=mux  block_config=sysgen:Mux_config
  Negate : hdlBasic/Negate  precision=Full  arith_type=Unsigned  n_bits=16  bin_pt=12  quantization=Truncate  overflow=Wrap  en=off  latency=0  XmcBlockStatus=1  maskContainerNames=tabcontainer1  block_type=negate  block_config=sysgen:Negate_config
  ROM : hdlBasic/ROM  depth=4  initVector=[1/3 1 -1/3 -1]  distributed_mem=Distributed memory  rst=off  init_reg=0  en=off  latency=0  gui_display_data_type=Fixed-point  arith_type="Signed  (2's comp)"  n_bits=16  bin_pt=15  preci_type=Single  exp_width=8  frac_width=24  optimize=Area  use_rpm=on  simulation_type=fast_sim  XmcBlockStatus=1  maskContainerNames=tabcontainer1  block_type=sprom  block_config=sysgen:SPROM_config
  Relational : hdlBasic/Relational  mode=a<b  op_type=Bool  en=off  latency=0  XmcBlockStatus=1  maskContainerNames=tabcontainer1  block_type=relational  block_config=sysgen:Relational_config
  Relational1 : hdlBasic/Relational  mode=a>=b  op_type=Bool  en=off  latency=0  XmcBlockStatus=1  maskContainerNames=tabcontainer1  block_type=relational  block_config=sysgen:Relational_config
  Slice : hdlBasic/Slice  nbits=1  boolean_output=off  mode=Upper Bit Location + Width  bit1=0  base1=MSB of Input  bit0=0  base0=LSB of Input  XmcBlockStatus=1  maskContainerNames=group1  block_type=slice  block_config=sysgen:Slice_config
  k1 : hdlBasic/Constant  const=2/3  gui_display_data_type=Fixed-point  arith_type=Unsigned  n_bits=8  bin_pt=8  preci_type=Single  exp_width=8  frac_width=24  explicit_period=off  period=1  XmcBlockStatus=1  maskContainerNames=tabcontainer1  block_type=constant  block_config=sysgen:Constant_config
  k2 : hdlBasic/Constant  const=0  gui_display_data_type=Fixed-point  arith_type=Unsigned  n_bits=8  bin_pt=0  preci_type=Single  exp_width=8  frac_width=24  explicit_period=off  period=1  XmcBlockStatus=1  maskContainerNames=tabcontainer1  block_type=constant  block_config=sysgen:Constant_config
  det : Outport  VectorParamsAs1DForOutWhenUnconnected=off
  wires:
  Slice/1 -> Mux/1
  x_n/1 -> Slice/1, Negate/1, Mux/2, Relational1/2
  Negate/1 -> Mux/3
  Mux/1 -> Relational/2
  k2/1 -> Relational1/1
  Relational/1 -> Concat/2
  Relational1/1 -> Concat/1
  Concat/1 -> ROM/1
  ROM/1 -> det/1
  k1/1 -> Relational/1

== system QAM16/DUT/Carrier Recovery/Phase Detector/Slicer/Q Map ==
  x_n : Inport
  Concat : hdlBasic/Concat  num_inputs=2  XmcBlockStatus=1  maskContainerNames=group1  block_type=concat  block_config=sysgen:Concat_config
  Mux : hdlBasic/Mux  inputs=2  en=off  latency=0  precision=Full  arith_type="Signed  (2's comp)"  n_bits=8  bin_pt=2  quantization=Truncate  overflow=Wrap  XmcBlockStatus=1  maskContainerNames=tabcontainer1  block_type=mux  block_config=sysgen:Mux_config
  Negate : hdlBasic/Negate  precision=Full  arith_type=Unsigned  n_bits=16  bin_pt=12  quantization=Truncate  overflow=Wrap  en=off  latency=0  XmcBlockStatus=1  maskContainerNames=tabcontainer1  block_type=negate  block_config=sysgen:Negate_config
  ROM : hdlBasic/ROM  depth=4  initVector=[1/3 1 -1/3 -1]  distributed_mem=Distributed memory  rst=off  init_reg=0  en=off  latency=0  gui_display_data_type=Fixed-point  arith_type="Signed  (2's comp)"  n_bits=16  bin_pt=15  preci_type=Single  exp_width=8  frac_width=24  optimize=Area  use_rpm=on  simulation_type=fast_sim  XmcBlockStatus=1  maskContainerNames=tabcontainer1  block_type=sprom  block_config=sysgen:SPROM_config
  Relational : hdlBasic/Relational  mode=a<b  op_type=Bool  en=off  latency=0  XmcBlockStatus=1  maskContainerNames=tabcontainer1  block_type=relational  block_config=sysgen:Relational_config
  Relational1 : hdlBasic/Relational  mode=a>=b  op_type=Bool  en=off  latency=0  XmcBlockStatus=1  maskContainerNames=tabcontainer1  block_type=relational  block_config=sysgen:Relational_config
  Slice : hdlBasic/Slice  nbits=1  boolean_output=off  mode=Upper Bit Location + Width  bit1=0  base1=MSB of Input  bit0=0  base0=LSB of Input  XmcBlockStatus=1  maskContainerNames=group1  block_type=slice  block_config=sysgen:Slice_config
  k1 : hdlBasic/Constant  const=2/3  gui_display_data_type=Fixed-point  arith_type=Unsigned  n_bits=8  bin_pt=8  preci_type=Single  exp_width=8  frac_width=24  explicit_period=off  period=1  XmcBlockStatus=1  maskContainerNames=tabcontainer1  block_type=constant  block_config=sysgen:Constant_config
  k2 : hdlBasic/Constant  const=0  gui_display_data_type=Fixed-point  arith_type=Unsigned  n_bits=8  bin_pt=0  preci_type=Single  exp_width=8  frac_width=24  explicit_period=off  period=1  XmcBlockStatus=1  maskContainerNames=tabcontainer1  block_type=constant  block_config=sysgen:Constant_config
  det : Outport  VectorParamsAs1DForOutWhenUnconnected=off
  wires:
  k1/1 -> Relational/1
  ROM/1 -> det/1
  Concat/1 -> ROM/1
  Relational1/1 -> Concat/1
  Relational/1 -> Concat/2
  k2/1 -> Relational1/1
  Mux/1 -> Relational/2
  Negate/1 -> Mux/3
  x_n/1 -> Relational1/2, Mux/2, Negate/1, Slice/1
  Slice/1 -> Mux/1

== system QAM16/DUT/Adaptive Equalizer/ALU/PE0/LMS Update/Cmplx Mult ==
  a_r : Inport
  a_i : Inport  Port=2
  b_r : Inport  Port=3
  b_i : Inport  Port=4
  AddSub : hdlBasic/AddSub  mode=Subtraction  use_carryin=off  use_carryout=off  en=off  latency=1  precision=User Defined  arith_type="Signed  (2's comp)"  n_bits=lms_mult_post_add_ni  bin_pt=lms_mult_post_add_nf  quantization=Truncate  overflow=Wrap  use_behavioral_HDL=on  hw_selection=Fabric  pipelined=off  use_rpm=on  XmcBlockStatus=1  maskContainerNames=tabcontainer1  block_type=addsub  block_config=sysgen:Addsub_config
  AddSub1 : hdlBasic/AddSub  mode=Addition  use_carryin=off  use_carryout=off  en=off  latency=1  precision=User Defined  arith_type="Signed  (2's comp)"  n_bits=lms_mult_post_add_ni  bin_pt=lms_mult_post_add_nf  quantization=Truncate  overflow=Wrap  use_behavioral_HDL=on  hw_selection=Fabric  pipelined=off  use_rpm=on  XmcBlockStatus=1  maskContainerNames=tabcontainer1  block_type=addsub  block_config=sysgen:Addsub_config
  Mult{1..4} (4 alike) : hdlBasic/Mult  precision=User Defined  arith_type="Signed  (2's comp)"  n_bits=lms_mult_ni  bin_pt=lms_mult_nf  quantization=Truncate  overflow=Wrap  en=off  latency=1  opt_float=off  fp_mult_usage=No Usage  use_behavioral_HDL=off  opt=Speed  use_embedded=on  optimum_pipeline=off  pipeline=off  use_rpm=on  placement_style=Rectangular shape  XmcBlockStatus=1  maskContainerNames=group1  block_type=mult  block_config=sysgen:Mult_config  block_width=598  block_height=876
  p_r : Outport  VectorParamsAs1DForOutWhenUnconnected=off
  p_i : Outport  Port=2  VectorParamsAs1DForOutWhenUnconnected=off
  wires:
  AddSub1/1 -> p_i/1
  AddSub/1 -> p_r/1
  Mult3/1 -> AddSub1/2
  Mult2/1 -> AddSub1/1
  Mult1/1 -> AddSub/2
  a_r/1 -> Mult2/1, Mult4/1
  b_i/1 -> Mult2/2, Mult1/2
  b_r/1 -> Mult3/1, Mult4/2
  a_i/1 -> Mult3/2, Mult1/1
  Mult4/1 -> AddSub/1
